simulink model "B_MotorSpeed"  (R2021b)
settings: Solver=VariableStepAuto  StartTime=0.0  StopTime=100  RelTol=1e-3
settings Model: Creator=vigne  LastModifiedBy=vigne

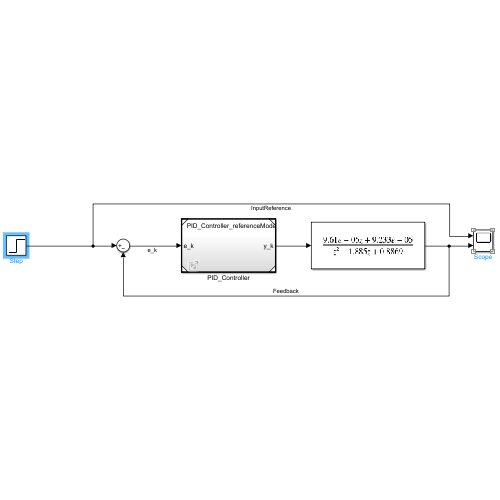
[thumbnail: Simulink's stored preview of the top-level diagram]
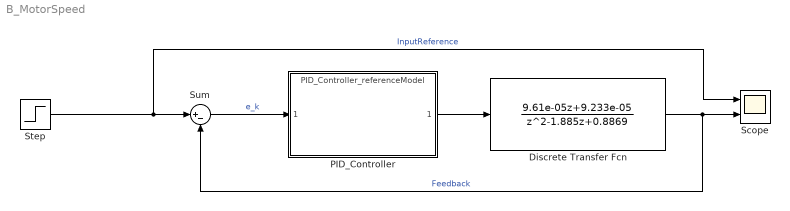
== system B_MotorSpeed ==
  Discrete Transfer Fcn : DiscreteTransferFcn  Numerator="[9.61e-05  9.233e-05]"  Denominator=[1 -1.885 0.8869]
  PID_Controller : ModelReference  ModelNameDialog=PID_Controller_referenceModel.slx  ModelReferenceVersion=1.6
  Scope : Scope  NumInputPorts=2
  Step : Step  After=100  SampleTime=0
  Sum : Sum  Inputs=|+-
  wires:
  PID_Controller/1 -> Discrete Transfer Fcn/1
  Sum/1 -> PID_Controller/1  "e_k"
  Step/1 -> Scope/1, Sum/1  "InputReference"
  Discrete Transfer Fcn/1 -> Sum/2, Scope/2  "Feedback"
